simulink model "TractionSystem"  (R2019b)
settings: configuration reference "ConfigSet_TractionSystem_Reference" (kept outside this file)
model workspace (MAT data in the model file):
  Prm_TractionSystem : Simulink.Parameter (value not decoded)
  SampleTime = 0.01
symbols that are objects in the model workspace (value not decoded): Prm_TractionSystem
undefined symbols (not defined in the file): Audio, BCU, Bogie, BogieNotIsolated, DiscIntNeverNeededParam, Dynamics, EDBrakeStatus, EDBrakingEffortAchieved, EDBrakingEffortPossible, ElectricalSystem, Forward, MaxAxles, Reverse, TCMS, TCUWheelSlideControlActive, TractionContactorStatus, TractionControl, TractionEDPower, Trafo_TCU, VehicleBogieDerailed, VehicleDerailed, WheelAngularVelocity
libraries: simulink x19, LatchesLib x3, TimersLib x2, WheelSlipControl_Lib x2, simulink_extras x2, TractionLib x2
(part 2 of 2)

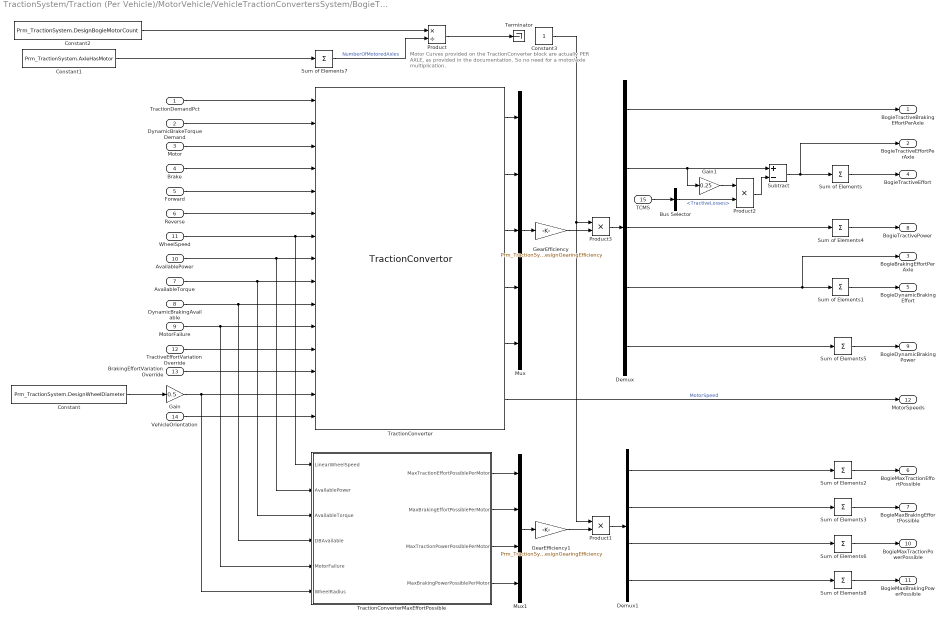
== system TractionSystem/Traction (Per Vehicle)/MotorVehicle/VehicleTractionConvertersSystem/BogieTractionConverterSystem (Per Bogie)/TractionConverterSystem ==
  note: Motor Curves provided on the TractionConverter block are actually PER AXLE, as provided in the documentation. So no need for a motor/axle multiplication.
  TractionDemandPct : Inport
  DynamicBrakeTorqueDemand : Inport  Port=2
  Motor : Inport  Port=3
  Brake : Inport  Port=4
  Forward : Inport  Port=5
  Reverse : Inport  Port=6
  AvailableTorque : Inport  Port=7
  DynamicBrakingAvailable : Inport  Port=8
  MotorFailure : Inport  Port=9
  AvailablePower : Inport  Port=10
  WheelSpeed : Inport  Port=11
  TractiveEffortVariationOverride : Inport  Port=12
  BrakingEffortVariationOverride : Inport  Port=13
  VehicleOrientation : Inport  Port=14
  TCMS : Inport  Port=15
  Bus Selector : BusSelector  OutputSignals=TractiveLosses
  Constant : Constant  Value=Prm_TractionSystem.DesignWheelDiameter
  Constant1 : Constant  Value=Prm_TractionSystem.AxleHasMotor
  Constant2 : Constant  Value=Prm_TractionSystem.DesignBogieMotorCount
  Constant3 : Constant
  Demux : Demux  Outputs=5
  Demux1 : Demux
  Gain : Gain  Gain=0.5
  Gain1 : Gain  Gain=0.25
  GearEfficiency : Gain  Gain=Prm_TractionSystem.DesignGearingEfficiency
  GearEfficiency1 : Gain  Gain=Prm_TractionSystem.DesignGearingEfficiency
  Mux : Mux  Inputs=5
  Mux1 : Mux
  Product : Product  Inputs=*/
  Product1 : Product  Inputs=**
  Product2 : Product
  Product3 : Product  Inputs=**
  Subtract : Sum  Inputs=+-
  Sum of Elements{,1..8} (9 alike) : Sum  Inputs=+
  Terminator : Terminator
  TractionConverter : TractionLib/TractionConvertor  TractionCurveInput=Curve Equations  TractionRatedTorque=Prm_TractionSystem.DesignMaxTractionTorque  TractionDesignPower=Prm_TractionSystem.DesignMaxTractionPower  TractionMotorSpeeds=[0 1]'  TractionMotorTorques=[34000 34000]'*(Prm_TractionSystem.DesignWheelDiameter/2)  VehicleTractionDataSize=2  CDMaxMotorTorque=Prm_TractionSystem.DesignMaxTractionTorque  CDMaxMotorPower=Prm_TractionSystem.DesignMaxTractionPower  TractionContourCount=4  TractionDemands=[1 2 3 4 0]  TractionDataSizes=[4 4 3 5 0]  TractionDataContours=permute(cat(3, [0 0; 1 1; 2 2; 3 3; 0 0;],[0 1; 1 2; 2.5 3; 5 4.5; 0 0;], [0 2; 2 4; 4 8; 0 0; 0 0;], [0 2.5; 1 4; 2 5; 3 9; 5 15;], [0 0; 0 0; 0 0; 0 0; 0 0;]), [3 2 1])  TractionMaximumTorques=[3 4.5 8 15 0]'  TractionMaximumPowers=[9 22.5 32 75 0]'  TractionRisingSlewRate=2e3  TractionFallingSlewRate=-5e3  BrakingCurveInput=Curve Equations  BrakingRatedTorque=Prm_TractionSystem.DesignMaxBrakingTorque  BrakingDesignPower=Prm_TractionSystem.DesignMaxBrakingPower  BrakingRampUpSpeeds=Prm_TractionSystem.BrakeFadeRampDownSpeeds  BrakingMotorSpeeds=[0 1]'  BrakingMotorTorques=[50000 50000]'*(Prm_TractionSystem.DesignWheelDiameter/2)  VehicleBrakingDataSize=2  BrakingDemands=[1 2 3 4 0]  BrakingDataSizes=[4 4 3 5 0]  BrakingDataContours=permute(cat(3, [0 0; 1 1; 2 2; 3 3; 0 0;],[0 1; 1 2; 2.5 3; 5 4.5; 0 0;], [0 2; 2 4; 4 8; 0 0; 0 0;], [0 2.5; 1 4; 2 5; 3 9; 5 15;], [0 0; 0 0; 0 0; 0 0; 0 0;]), [3 2 1])  BrakingRisingSlewRate=5e3  BrakingFallingSlewRate=-5e3  AxleHasMotor=Prm_TractionSystem.AxleHasMotor  GearRatio=Prm_TractionSystem.DesignGearingRatio
      settings: SourceProductName=Train Utilities
  TractionConverterMaxEffortPossible : Subsystem  mask{TractionRatedTorque=Prm_TractionSystem.DesignMaxTractionTorque, TractionDesignPower=Prm_TractionSystem.DesignMaxTractionPower, BrakingRatedTorque=Prm_TractionSystem.DesignMaxBrakingTorque, BrakingDesignPower=Prm_TractionSystem.DesignMaxBrakingPower, RampUpSpeeds=Prm_TractionSystem.BrakeFadeRampDownSpeeds, AxleHasMotor=Prm_TractionSystem.AxleHasMotor, GearRatio=Prm_TractionSystem.DesignGearingRatio}
      mask prompts: TractionRatedTorque "This is the constant torque for 1 motor (removing design gearing ratio and wheel diameter factors) [Nm]:"; TractionDesignPower "This is the Constant power for 100% Demand (and should be Rated Torque* Corner Motor Speed) [Nm/s]:"; BrakingRatedTorque "This is the constant torque for 1 motor (removing design gearing ratio and wheel diameter factors) [Nm]:"; BrakingDesignPower "This is the constant power for 100% Demand (and should be Rated Torque* Corner Motor Speed) [Nm/s]:"; RampUpSpeeds "This is a list of the two motor speeds between which the Dynamic Braking Avilable is ramped between 0 and 100% [rad/s]:"; GearRatio "Gear Ratio"
      mask DialogControl TractionParam Prompt: Traction
      mask DialogControl Container11 Prompt: Braking
      mask DialogControl Container9 Prompt: General
      mask DialogControl GearParam Prompt: Gearing
  BogieTractiveBrakingEffortPerAxle : Outport  PortDimensions=2
  BogieTractiveEffortPerAxle : Outport  Port=2  PortDimensions=2
  BogieBrakingEffortPerAxle : Outport  Port=3  PortDimensions=2
  BogieTractiveEffort : Outport  Port=4
  BogieDynamicBrakingEffort : Outport  Port=5
  BogieMaxTractionEffortPossible : Outport  Port=6
  BogieMaxBrakingEffortPossible : Outport  Port=7
  BogieTractivePower : Outport  Port=8
  BogieDynamicBrakingPower : Outport  Port=9
  BogieMaxTractionPowerPossible : Outport  Port=10
  BogieMaxBrakingPowerPossible : Outport  Port=11
  MotorSpeeds : Outport  Port=12
  wires:
  AvailablePower/1 -> TractionConverterMaxEffortPossible/2(AvailablePower), TractionConverter/8
  BrakingEffortVariationOverride/1 -> TractionConverter/13
  VehicleOrientation/1 -> TractionConverter/15
  MotorFailure/1 -> TractionConverterMaxEffortPossible/5(MotorFailure), TractionConverter/11
  TractiveEffortVariationOverride/1 -> TractionConverter/12
  DynamicBrakingAvailable/1 -> TractionConverterMaxEffortPossible/4(DBAvailable), TractionConverter/10
  AvailableTorque/1 -> TractionConverterMaxEffortPossible/3(AvailableTorque), TractionConverter/9
  TractionConverter/6 -> MotorSpeeds/1  "MotorSpeed"
  Constant/1 -> Gain/1
  TractionDemandPct/1 -> TractionConverter/1
  DynamicBrakeTorqueDemand/1 -> TractionConverter/2
  Motor/1 -> TractionConverter/3
  Brake/1 -> TractionConverter/4
  Forward/1 -> TractionConverter/5
  Reverse/1 -> TractionConverter/6
  WheelSpeed/1 -> TractionConverterMaxEffortPossible/1(LinearWheelSpeed), TractionConverter/7
  Sum of Elements/1 -> BogieTractiveEffort/1
  Sum of Elements1/1 -> BogieDynamicBrakingEffort/1
  Gain/1 -> TractionConverterMaxEffortPossible/6(WheelRadius), TractionConverter/14
  TractionConverterMaxEffortPossible/1(MaxTractionEffortPossiblePerMotor) -> Mux1/1
  TractionConverterMaxEffortPossible/2(MaxBrakingEffortPossiblePerMotor) -> Mux1/2
  Sum of Elements2/1 -> BogieMaxTractionEffortPossible/1
  Sum of Elements3/1 -> BogieMaxBrakingEffortPossible/1
  Sum of Elements4/1 -> BogieTractivePower/1
  Sum of Elements5/1 -> BogieDynamicBrakingPower/1
  Constant1/1 -> Sum of Elements7/1
  Sum of Elements7/1 -> Product/2  "NumberOfMotoredAxles"
  Constant2/1 -> Product/1
  Subtract/1 -> BogieTractiveEffortPerAxle/1, Sum of Elements/1
  Demux/3 -> Sum of Elements4/1
  Demux/5 -> Sum of Elements5/1
  TractionConverter/1 -> Mux/1
  TractionConverter/2 -> Mux/2
  TractionConverter/3 -> Mux/3
  TractionConverter/4 -> Mux/4
  TractionConverter/5 -> Mux/5
  Mux/1 -> GearEfficiency/1
  GearEfficiency/1 -> Product3/2
  Product3/1 -> Demux/1
  Demux/1 -> BogieTractiveBrakingEffortPerAxle/1
  Product1/1 -> Demux1/1
  Constant3/1 -> Product1/1, Product3/1
  GearEfficiency1/1 -> Product1/2
  Mux1/1 -> GearEfficiency1/1
  Demux1/1 -> Sum of Elements2/1
  Demux1/2 -> Sum of Elements3/1
  Product/1 -> Terminator/1
  TractionConverterMaxEffortPossible/3(MaxTractionPowerPossiblePerMotor) -> Mux1/3
  TractionConverterMaxEffortPossible/4(MaxBrakingPowerPossiblePerMotor) -> Mux1/4
  Demux1/4 -> Sum of Elements8/1
  Demux1/3 -> Sum of Elements6/1
  Sum of Elements8/1 -> BogieMaxBrakingPowerPossible/1
  Sum of Elements6/1 -> BogieMaxTractionPowerPossible/1
  Demux/4 -> BogieBrakingEffortPerAxle/1, Sum of Elements1/1
  TCMS/1 -> Bus Selector/1
  Bus Selector/1 -> Product2/2  "<TractiveLosses>"
  Demux/2 -> Gain1/1, Subtract/1
  Product2/1 -> Subtract/2
  Gain1/1 -> Product2/1

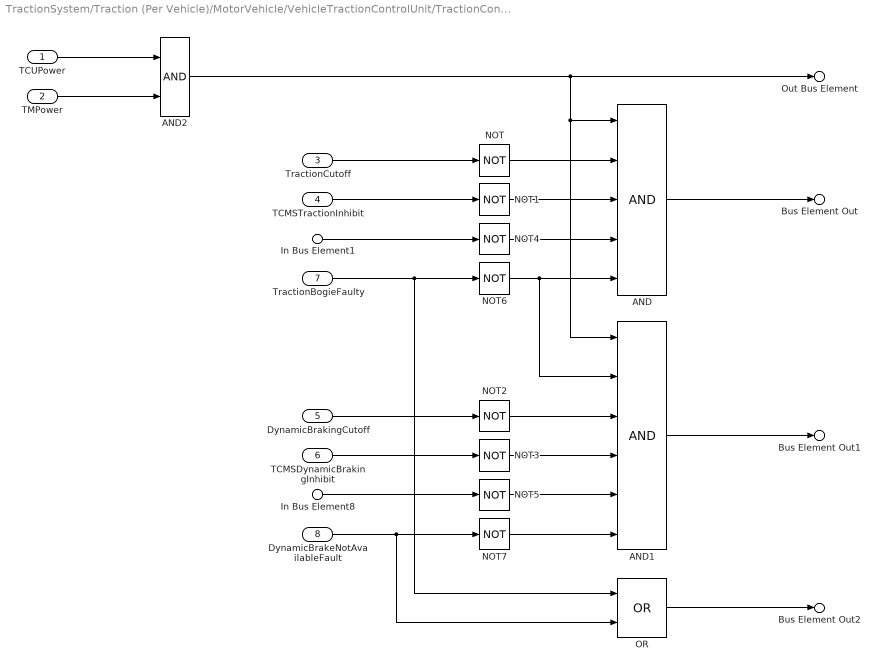
== system TractionSystem/Traction (Per Vehicle)/MotorVehicle/VehicleTractionControlUnit/TractionControl (Per Bogie)/TCUONLogic/BogieTractionBrakingAvailable ==
  TCUPower : Inport
  TMPower : Inport  Port=2
  TractionCutoff : Inport  Port=3
  TCMSTractionInhibit : Inport  Port=4
  DynamicBrakingCutoff : Inport  Port=5
  TCMSDynamicBrakingInhibit : Inport  Port=6
  TractionBogieFaulty : Inport  Port=7
  DynamicBrakeNotAvailableFault : Inport  Port=8
  In Bus Element8 : Inport  Port=9  PortName=WheelSlipSlideProtection  Element=WSPBrakeCutOut
  In Bus Element1 : Inport  Port=9  PortName=WheelSlipSlideProtection  Element=WSPTractionCutOut
  AND : Logic  Inputs=5  AllPortsSameDT=off  OutDataTypeStr=boolean
  AND1 : Logic  Inputs=6  AllPortsSameDT=off  OutDataTypeStr=boolean
  AND2 : Logic  AllPortsSameDT=off  OutDataTypeStr=boolean
  NOT{,1..7} (8 alike) : Logic  Operator=NOT  AllPortsSameDT=off  OutDataTypeStr=boolean
  OR : Logic  Operator=OR  AllPortsSameDT=off  OutDataTypeStr=boolean
  Bus Element Out : Outport  PortName=TCStatuses  Element=TractionAvailable
  Bus Element Out1 : Outport  PortName=TCStatuses  Element=EDBrakeAvailable
  Out Bus Element : Outport  PortName=TCStatuses  Element=TCUResponseStatus
  Bus Element Out2 : Outport  PortName=TCStatuses  Element=BogieFaulty
  wires:
  AND/1 -> Bus Element Out/1
  AND1/1 -> Bus Element Out1/1
  AND2/1 -> AND1/1, AND/1, Out Bus Element/1
  TractionCutoff/1 -> NOT/1
  NOT/1 -> AND/2
  TCMSTractionInhibit/1 -> NOT1/1
  NOT1/1 -> AND/3
  TCMSDynamicBrakingInhibit/1 -> NOT3/1
  DynamicBrakingCutoff/1 -> NOT2/1
  NOT3/1 -> AND1/4
  NOT2/1 -> AND1/3
  In Bus Element1/1 -> NOT4/1
  NOT4/1 -> AND/4
  In Bus Element8/1 -> NOT5/1
  NOT5/1 -> AND1/5
  TractionBogieFaulty/1 -> OR/1, NOT6/1
  NOT6/1 -> AND/5, AND1/2
  DynamicBrakeNotAvailableFault/1 -> OR/2, NOT7/1
  NOT7/1 -> AND1/6
  OR/1 -> Bus Element Out2/1
  TMPower/1 -> AND2/2
  TCUPower/1 -> AND2/1

== system TractionSystem/Traction (Per Vehicle)/MotorVehicle/VehicleTractionControlUnit/TractionControl (Per Bogie)/TCUONLogic/DirectionControl ==
  Forward : Inport
  Reverse : Inport  Port=2
  AND : Logic  AllPortsSameDT=off  OutDataTypeStr=boolean
  AND1 : Logic  AllPortsSameDT=off  OutDataTypeStr=boolean
  NOT : Logic  Operator=NOT  AllPortsSameDT=off  OutDataTypeStr=boolean
  NOT1 : Logic  Operator=NOT  AllPortsSameDT=off  OutDataTypeStr=boolean
  Bus Element Out : Outport  PortName=DirectionControl  Element=Forward
  Bus Element Out1 : Outport  PortName=DirectionControl  Element=Reverse
  wires:
  Reverse/1 -> NOT1/1, AND/2  "Reverse"
  Forward/1 -> AND1/1, NOT/1  "Forward"
  NOT/1 -> AND/1
  NOT1/1 -> AND1/2
  AND1/1 -> Bus Element Out/1
  AND/1 -> Bus Element Out1/1

== system TractionSystem/Traction (Per Vehicle)/MotorVehicle/VehicleTractionControlUnit/TractionControl (Per Bogie)/TCUONLogic/TCUControlsAssign ==
  In Bus Element : Inport  PortName=DirectionControl  Element=Forward
  In Bus Element1 : Inport  PortName=DirectionControl  Element=Reverse
  Bus Element In : Inport  Port=2  PortName=TCUStatuses  Element=TractionAvailable
  In Bus Element9 : Inport  Port=2  PortName=TCUStatuses  Element=EDBrakeAvailable
  In Bus Element2 : Inport  Port=3  PortName=TRBCommands  Element=BrakingTorqueDemand
  In Bus Element3 : Inport  Port=3  PortName=TRBCommands  Element=TractionDemandPct
  In Bus Element4 : Inport  Port=4  PortName=TRBInterlocks  Element=TractionInterlock
  In Bus Element5 : Inport  Port=4  PortName=TRBInterlocks  Element=BrakingInterlock
  Bus Creator : BusCreator  Inputs=9  OutDataTypeStr=Bus: BD_TractionSystem_Int_BogieControl  NonVirtualBus=on
  Constant1 : Constant  Value=Prm_TractionSystem.AxleHasMotor
  Data Type Conversion{1..9} (9 alike) : DataTypeConversion
  Data Type Conversion10 : DataTypeConversion  OutDataTypeStr=double
  NOT1 : Logic  Operator=NOT  AllPortsSameDT=off  OutDataTypeStr=boolean
  Product : Product
  TractionControlOut : Outport
  wires:
  Data Type Conversion6/1 -> Bus Creator/8  "TractionTorqueAvailable"
  In Bus Element4/1 -> Data Type Conversion2/1
  Data Type Conversion1/1 -> Bus Creator/4  "Braking"
  Data Type Conversion8/1 -> Bus Creator/9  "DynamicBrakeAvailable"
  Constant1/1 -> Product/1
  Data Type Conversion2/1 -> Bus Creator/3  "Powering"
  Bus Element In/1 -> Data Type Conversion6/1, Data Type Conversion10/1
  In Bus Element5/1 -> Data Type Conversion1/1
  Bus Creator/1 -> TractionControlOut/1
  In Bus Element3/1 -> Data Type Conversion9/1
  In Bus Element2/1 -> Data Type Conversion7/1
  In Bus Element1/1 -> Data Type Conversion4/1
  Data Type Conversion4/1 -> Bus Creator/6  "Reverse"
  Data Type Conversion3/1 -> Bus Creator/5  "Forward"
  In Bus Element/1 -> Data Type Conversion3/1
  NOT1/1 -> Data Type Conversion5/1
  Data Type Conversion5/1 -> Bus Creator/7  "MotorNotAvailable"
  Product/1 -> NOT1/1
  Data Type Conversion10/1 -> Product/2
  In Bus Element9/1 -> Data Type Conversion8/1
  Data Type Conversion7/1 -> Bus Creator/2  "DynamicBrakeTorqueDemand"
  Data Type Conversion9/1 -> Bus Creator/1  "TractionDemandPct"

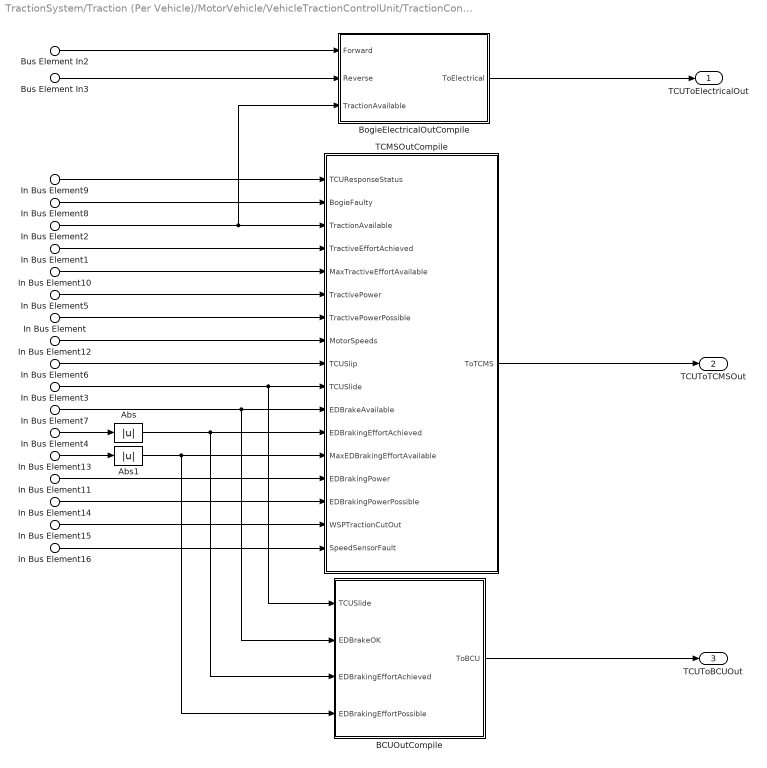
== system TractionSystem/Traction (Per Vehicle)/MotorVehicle/VehicleTractionControlUnit/TractionControl (Per Bogie)/TCUONLogic/TCUOutputsAssign ==
  Bus Element In2 : Inport  PortName=DirectionControlOut  Element=Forward
  Bus Element In3 : Inport  PortName=DirectionControlOut  Element=Reverse
  In Bus Element1 : Inport  Port=2  PortName=TractionConverterOut  Element=BogieTractiveEffort
  In Bus Element4 : Inport  Port=2  PortName=TractionConverterOut  Element=BogieDynamicBrakingEffort
  In Bus Element10 : Inport  Port=2  PortName=TractionConverterOut  Element=BogieMaxTractionEffortPossible
  In Bus Element5 : Inport  Port=2  PortName=TractionConverterOut  Element=BogieTractivePower
  In Bus Element11 : Inport  Port=2  PortName=TractionConverterOut  Element=BogieDynamicBrakingPower
  In Bus Element12 : Inport  Port=2  PortName=TractionConverterOut  Element=BogieMotorSpeeds
  In Bus Element13 : Inport  Port=2  PortName=TractionConverterOut  Element=BogieMaxBrakingEffortPossible
  In Bus Element : Inport  Port=2  PortName=TractionConverterOut  Element=BogieMaxTractionPowerPossible
  In Bus Element14 : Inport  Port=2  PortName=TractionConverterOut  Element=BogieMaxBrakingPowerPossible
  In Bus Element2 : Inport  Port=3  PortName=TCStatuses  Element=TractionAvailable
  In Bus Element7 : Inport  Port=3  PortName=TCStatuses  Element=EDBrakeAvailable
  In Bus Element9 : Inport  Port=3  PortName=TCStatuses  Element=TCUResponseStatus
  In Bus Element8 : Inport  Port=3  PortName=TCStatuses  Element=BogieFaulty
  In Bus Element3 : Inport  Port=4  PortName=WheelSlipSlideProtection  Element=TCUSlide
  In Bus Element6 : Inport  Port=4  PortName=WheelSlipSlideProtection  Element=TCUSlip
  In Bus Element15 : Inport  Port=4  PortName=WheelSlipSlideProtection  Element=WSPTractionCutOut
  In Bus Element16 : Inport  Port=5  PortName=Sensor  Element=SpeedSensorFault
  Abs : Abs
  Abs1 : Abs
  BCUOutCompile : Subsystem
  BogieElectricalOutCompile : Subsystem
  TCMSOutCompile : Subsystem
  TCUToElectricalOut : Outport
  TCUToTCMSOut : Outport  Port=2
  TCUToBCUOut : Outport  Port=3
  wires:
  TCMSOutCompile/1(ToTCMS) -> TCUToTCMSOut/1
  In Bus Element7/1 -> BCUOutCompile/2(EDBrakeOK), TCMSOutCompile/11(EDBrakeAvailable)
  In Bus Element4/1 -> Abs/1
  In Bus Element1/1 -> TCMSOutCompile/4(TractiveEffortAchieved)
  BCUOutCompile/1(ToBCU) -> TCUToBCUOut/1
  BogieElectricalOutCompile/1(ToElectrical) -> TCUToElectricalOut/1
  In Bus Element10/1 -> TCMSOutCompile/5(MaxTractiveEffortAvailable)
  In Bus Element13/1 -> Abs1/1
  In Bus Element3/1 -> BCUOutCompile/1(TCUSlide), TCMSOutCompile/10(TCUSlide)
  Bus Element In2/1 -> BogieElectricalOutCompile/1(Forward)
  In Bus Element2/1 -> BogieElectricalOutCompile/3(TractionAvailable), TCMSOutCompile/3(TractionAvailable)
  In Bus Element6/1 -> TCMSOutCompile/9(TCUSlip)
  Abs/1 -> BCUOutCompile/3(EDBrakingEffortAchieved), TCMSOutCompile/12(EDBrakingEffortAchieved)
  Abs1/1 -> BCUOutCompile/4(EDBrakingEffortPossible), TCMSOutCompile/13(MaxEDBrakingEffortAvailable)
  In Bus Element9/1 -> TCMSOutCompile/1(TCUResponseStatus)
  Bus Element In3/1 -> BogieElectricalOutCompile/2(Reverse)
  In Bus Element11/1 -> TCMSOutCompile/14(EDBrakingPower)
  In Bus Element5/1 -> TCMSOutCompile/6(TractivePower)
  In Bus Element12/1 -> TCMSOutCompile/8(MotorSpeeds)
  In Bus Element/1 -> TCMSOutCompile/7(TractivePowerPossible)
  In Bus Element14/1 -> TCMSOutCompile/15(EDBrakingPowerPossible)
  In Bus Element8/1 -> TCMSOutCompile/2(BogieFaulty)
  In Bus Element15/1 -> TCMSOutCompile/16(WSPTractionCutOut)
  In Bus Element16/1 -> TCMSOutCompile/17(SpeedSensorFault)

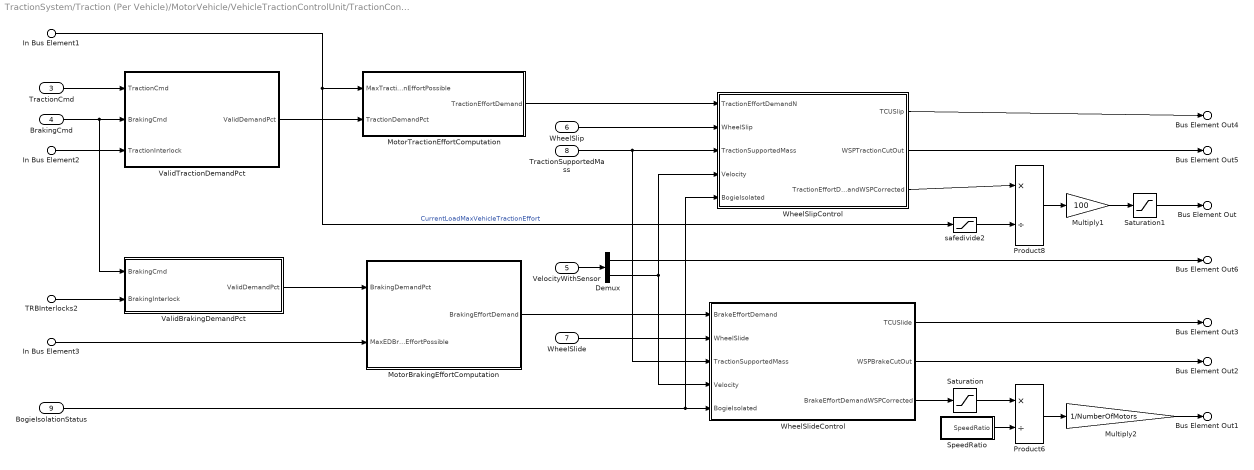
== system TractionSystem/Traction (Per Vehicle)/MotorVehicle/VehicleTractionControlUnit/TractionControl (Per Bogie)/TCUONLogic/TractionBrakingDemandControl ==
  In Bus Element1 : Inport  PortName=TCOut  Element=BogieMaxTractionEffortPossible
  In Bus Element3 : Inport  PortName=TCOut  Element=BogieMaxBrakingEffortPossible
  TRBInterlocks2 : Inport  Port=2  PortName=TRBInterlocks  Element=BrakingInterlock
  In Bus Element2 : Inport  Port=2  PortName=TRBInterlocks  Element=TractionInterlock
  TractionCmd : Inport  Port=3
  BrakingCmd : Inport  Port=4
  VelocityWithSensor : Inport  Port=5
  WheelSlip : Inport  Port=6
  WheelSlide : Inport  Port=7
  TractionSupportedMass : Inport  Port=8
  BogieIsolationStatus : Inport  Port=9
  Demux : Demux  Outputs=2
  MotorBrakingEffortComputation : Subsystem
  MotorTractionEffortComputation : Subsystem
  Multiply1 : Gain  Gain=100
  Multiply2 : Gain  Gain=1/NumberOfMotors
  Product6 : Product  Inputs=*/
  Product8 : Product  Inputs=*/
  Saturation : Saturate  UpperLimit=inf  LowerLimit=0
  Saturation1 : Saturate  UpperLimit=100  LowerLimit=0
  SpeedRatio : Subsystem
  ValidBrakingDemandPct : Subsystem
  ValidTractionDemandPct : Subsystem
  WheelSlideControl : Subsystem
  WheelSlipControl : Subsystem
  safedivide2 : Saturate  UpperLimit=1e8  LowerLimit=eps
  Bus Element Out2 : Outport  PortName=WheelSlipSlideProtection  Element=WSPBrakeCutOut
  Bus Element Out3 : Outport  PortName=WheelSlipSlideProtection  Element=TCUSlide
  Bus Element Out4 : Outport  PortName=WheelSlipSlideProtection  Element=TCUSlip
  Bus Element Out5 : Outport  PortName=WheelSlipSlideProtection  Element=WSPTractionCutOut
  Bus Element Out6 : Outport  Port=2  PortName=Sensor  Element=SpeedSensorFault
  Bus Element Out : Outport  Port=3  PortName=TRBCommands  Element=TractionDemandPct
  Bus Element Out1 : Outport  Port=3  PortName=TRBCommands  Element=BrakingTorqueDemand
  wires:
  Product8/1 -> Multiply1/1
  Product6/1 -> Multiply2/1
  Saturation/1 -> Product6/1
  WheelSlideControl/3(BrakeEffortDemandWSPCorrected) -> Saturation/1
  MotorTractionEffortComputation/1(TractionEffortDemand) -> WheelSlipControl/1(TractionEffortDemandN)
  SpeedRatio/1(SpeedRatio) -> Product6/2
  WheelSlide/1 -> WheelSlideControl/2(WheelSlide)
  WheelSlideControl/2(WSPBrakeCutOut) -> Bus Element Out2/1
  WheelSlideControl/1(TCUSlide) -> Bus Element Out3/1
  WheelSlipControl/1("TCUSlip ") -> Bus Element Out4/1
  WheelSlip/1 -> WheelSlipControl/2(WheelSlip)
  WheelSlipControl/3(TractionEffortDemandWSPCorrected) -> Product8/1
  In Bus Element1/1 -> safedivide2/1, MotorTractionEffortComputation/1(MaxTractionEffortPossible)  "CurrentLoadMaxVehicleTractionEffort"
  Multiply1/1 -> Saturation1/1
  BrakingCmd/1 -> ValidTractionDemandPct/2(BrakingCmd), ValidBrakingDemandPct/1(BrakingCmd)
  ValidBrakingDemandPct/1(ValidDemandPct) -> MotorBrakingEffortComputation/1(BrakingDemandPct)
  TractionCmd/1 -> ValidTractionDemandPct/1(TractionCmd)
  ValidTractionDemandPct/1(ValidDemandPct) -> MotorTractionEffortComputation/2(TractionDemandPct)
  MotorBrakingEffortComputation/1(BrakingEffortDemand) -> WheelSlideControl/1(BrakeEffortDemand)
  safedivide2/1 -> Product8/2
  Saturation1/1 -> Bus Element Out/1
  In Bus Element3/1 -> MotorBrakingEffortComputation/2(MaxEDBrakingEffortPossible)
  In Bus Element2/1 -> ValidTractionDemandPct/3(TractionInterlock)
  TRBInterlocks2/1 -> ValidBrakingDemandPct/2(BrakingInterlock)
  TractionSupportedMass/1 -> WheelSlideControl/3(TractionSupportedMass), WheelSlipControl/3(TractionSupportedMass)
  Multiply2/1 -> Bus Element Out1/1
  WheelSlipControl/2(WSPTractionCutOut) -> Bus Element Out5/1
  Demux/2 -> WheelSlipControl/4(Velocity), WheelSlideControl/4(Velocity)
  VelocityWithSensor/1 -> Demux/1
  Demux/1 -> Bus Element Out6/1
  BogieIsolationStatus/1 -> WheelSlipControl/5(BogieIsolated), WheelSlideControl/5(BogieIsolated)

== system TractionSystem/Traction (Per Vehicle)/MotorVehicle/VehicleTractionControlUnit/TractionControl (Per Bogie)/TCUONLogic/TractionBrakingInterlocks ==
  Bus Element In2 : Inport  PortName=DirectionControlOut  Element=Forward
  Bus Element In3 : Inport  PortName=DirectionControlOut  Element=Reverse
  TractionAuthorisation : Inport  Port=2
  TractionActive : Inport  Port=3
  NoEmergencyBrakeActive : Inport  Port=4
  Constant : Constant  Value=true  OutDataTypeStr=boolean
  Constant1 : Constant  Value=EBdeactivateED
  Data Type Conversion3 : DataTypeConversion
  Data Type Conversion4 : DataTypeConversion
  OR1 : Logic  Operator=OR  AllPortsSameDT=off  OutDataTypeStr=boolean
  Switch : Switch  Criteria=u2 > Threshold
  Vector Concatenate : Concatenate  NumInputs=3
  Vector Concatenate1 : Concatenate
  and : Logic  AllPortsSameDT=off  OutDataTypeStr=boolean
  and1 : Logic  Inputs=1  AllPortsSameDT=off  OutDataTypeStr=boolean
  and5 : Logic  Inputs=1  AllPortsSameDT=off  OutDataTypeStr=boolean
  Bus Element Out : Outport  PortName=TRBInterlocks  Element=TractionInterlock
  Bus Element Out1 : Outport  PortName=TRBInterlocks  Element=BrakingInterlock
  wires:
  and/1 -> Data Type Conversion3/1
  Data Type Conversion3/1 -> Bus Element Out/1  "TractionInterlock"
  Data Type Conversion4/1 -> Bus Element Out1/1  "BrakingInterlock"
  and1/1 -> and/1, Data Type Conversion4/1
  Vector Concatenate/1 -> and5/1
  Bus Element In2/1 -> OR1/1
  Bus Element In3/1 -> OR1/2
  OR1/1 -> Vector Concatenate1/1
  TractionActive/1 -> Vector Concatenate/2
  NoEmergencyBrakeActive/1 -> Switch/1, Vector Concatenate/1
  and5/1 -> and/2
  Vector Concatenate1/1 -> and1/1
  Switch/1 -> Vector Concatenate1/2
  Constant/1 -> Switch/3
  Constant1/1 -> Switch/2
  TractionAuthorisation/1 -> Vector Concatenate/3

== system TractionSystem/Traction (Per Vehicle)/MotorVehicle/VehicleTractionConvertersSystem/BogieTractionConverterSystem (Per Bogie)/TractionConverterSystem/TractionConverterMaxEffortPossible ==
  LinearWheelSpeed : Inport
  AvailablePower : Inport  Port=2
  AvailableTorque : Inport  Port=3
  DBAvailable : Inport  Port=4
  MotorFailure : Inport  Port=5
  WheelRadius : Inport  Port=6
  Assignment : Assignment  DiagnosticForDimensions=Warning  IndexOptions=Assign all  Indices=1  OutputSizes=1
  Constant : Constant  Value=AxleHasMotor
  MotorVehicle : Subsystem
  MaxTractionEffortPossiblePerMotor : Outport
  MaxBrakingEffortPossiblePerMotor : Outport  Port=2
  MaxTractionPowerPossiblePerMotor : Outport  Port=3
  MaxBrakingPowerPossiblePerMotor : Outport  Port=4
  wires:
  LinearWheelSpeed/1 -> Assignment/2
  AvailablePower/1 -> MotorVehicle/3(AvailablePower)
  AvailableTorque/1 -> MotorVehicle/4(AvailableTorque)
  WheelRadius/1 -> MotorVehicle/5(WheelRadius)
  MotorVehicle/1(MaximumTractionEffortPossible) -> MaxTractionEffortPossiblePerMotor/1
  MotorVehicle/2(MaxBrakingEffortPossible) -> MaxBrakingEffortPossiblePerMotor/1
  Constant/1 -> Assignment/1, MotorVehicle/1(AxleHasMotor)
  MotorFailure/1 -> MotorVehicle/6(MotorFailure)
  DBAvailable/1 -> MotorVehicle/7(DBAvailable)
  MotorVehicle/4(MaxBrakingPowerPossible) -> MaxBrakingPowerPossiblePerMotor/1
  MotorVehicle/3(MaxTractionPowerPossible) -> MaxTractionPowerPossiblePerMotor/1
  Assignment/1 -> MotorVehicle/2(LinearWheelSpeed)

== system TractionSystem/Traction (Per Vehicle)/MotorVehicle/VehicleTractionControlUnit/TractionControl (Per Bogie)/TCUONLogic/TCUOutputsAssign/BCUOutCompile ==
  TCUSlide : Inport
  EDBrakeOK : Inport  Port=2
  EDBrakingEffortAchieved : Inport  Port=3
  EDBrakingEffortPossible : Inport  Port=4
  Bus Assignment1 : BusAssignment  AssignedSignals=TCUWheelSlideControlActive,EDBrakeStatus,EDBrakingEffortAchieved,EDBrakingEffortPossible
  Constant1 : Constant  Value=0  OutDataTypeStr=Bus: BD_TractionSystem_Out_Vehicle_BCU_Bogie
  Data Type Conversion : DataTypeConversion
  ToBCU : Outport
  wires:
  Bus Assignment1/1 -> ToBCU/1  "ToBCU"
  Constant1/1 -> Bus Assignment1/1
  EDBrakeOK/1 -> Bus Assignment1/3
  EDBrakingEffortPossible/1 -> Bus Assignment1/5  "TotalEDBrakingEffortPossible"
  EDBrakingEffortAchieved/1 -> Bus Assignment1/4  "TotalEDBrakingEffortAchieved"
  TCUSlide/1 -> Data Type Conversion/1
  Data Type Conversion/1 -> Bus Assignment1/2

== system TractionSystem/Traction (Per Vehicle)/MotorVehicle/VehicleTractionControlUnit/TractionControl (Per Bogie)/TCUONLogic/TCUOutputsAssign/BogieElectricalOutCompile ==
  Forward : Inport
  Reverse : Inport  Port=2
  TractionAvailable : Inport  Port=3
  Bus Assignment1 : BusAssignment  AssignedSignals=Forward,Reverse,BogieNotIsolated
  Constant4 : Constant  Value=0  OutDataTypeStr=Bus: BD_TractionSystem_Out_Vehicle_ElectricalSystem_Bogie
  Data Type Conversion : DataTypeConversion  OutDataTypeStr=boolean
  Data Type Conversion1 : DataTypeConversion  OutDataTypeStr=boolean
  Data Type Conversion2 : DataTypeConversion  OutDataTypeStr=boolean
  ToElectrical : Outport
  wires:
  Reverse/1 -> Data Type Conversion1/1
  Forward/1 -> Data Type Conversion/1
  Constant4/1 -> Bus Assignment1/1
  Bus Assignment1/1 -> ToElectrical/1  "ToElectrical"
  TractionAvailable/1 -> Data Type Conversion2/1
  Data Type Conversion/1 -> Bus Assignment1/2
  Data Type Conversion1/1 -> Bus Assignment1/3
  Data Type Conversion2/1 -> Bus Assignment1/4

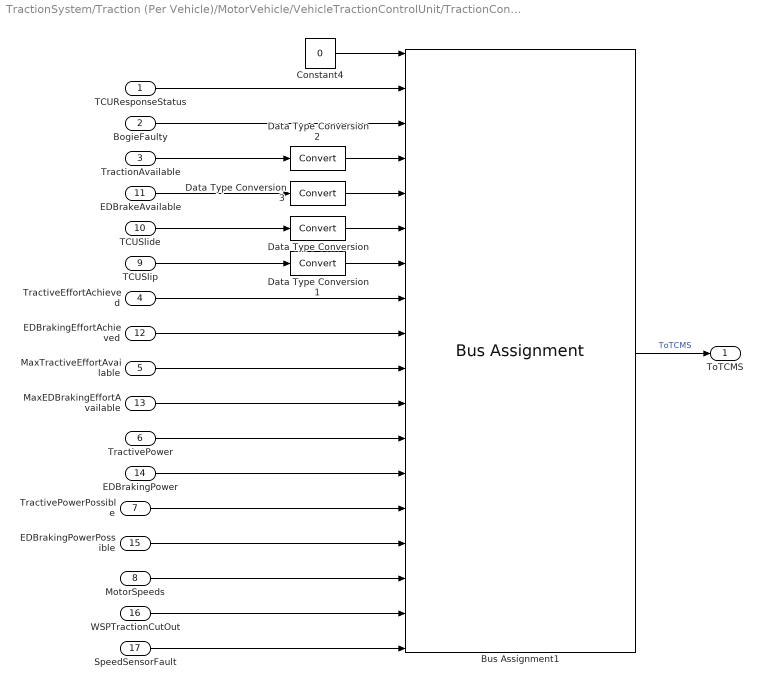
== system TractionSystem/Traction (Per Vehicle)/MotorVehicle/VehicleTractionControlUnit/TractionControl (Per Bogie)/TCUONLogic/TCUOutputsAssign/TCMSOutCompile ==
  TCUResponseStatus : Inport
  BogieFaulty : Inport  Port=2
  TractionAvailable : Inport  Port=3
  TractiveEffortAchieved : Inport  Port=4
  MaxTractiveEffortAvailable : Inport  Port=5
  TractivePower : Inport  Port=6
  TractivePowerPossible : Inport  Port=7
  MotorSpeeds : Inport  Port=8
  TCUSlip : Inport  Port=9
  TCUSlide : Inport  Port=10
  EDBrakeAvailable : Inport  Port=11
  EDBrakingEffortAchieved : Inport  Port=12
  MaxEDBrakingEffortAvailable : Inport  Port=13
  EDBrakingPower : Inport  Port=14
  EDBrakingPowerPossible : Inport  Port=15
  WSPTractionCutOut : Inport  Port=16
  SpeedSensorFault : Inport  Port=17
  Bus Assignment1 : BusAssignment  AssignedSignals=TCUStatus,BogieFaulty,TractionNotIsolated,EDBrakeNotIsolated,TCUSlideDetected,TCUSlipDetected,TractiveEffortAchieved,EDBrakingEffortAchieved,TractiveEffortPossible,EDBrakingEffortPossible,TractionPower,EDBrakingPower,TractivePowerPossible,EDBrakingPowerPossible,MotorSpeeds,WSPTractionCutout,SpeedSensorFault
  Constant4 : Constant  Value=0  OutDataTypeStr=Bus: BD_TractionSystem_Out_Vehicle_TCMS_Bogie
  Data Type Conversion{,1..3} (4 alike) : DataTypeConversion
  ToTCMS : Outport
  wires:
  TCUSlide/1 -> Data Type Conversion/1
  Bus Assignment1/1 -> ToTCMS/1  "ToTCMS"
  Constant4/1 -> Bus Assignment1/1
  TCUSlip/1 -> Data Type Conversion1/1
  TCUResponseStatus/1 -> Bus Assignment1/2
  TractionAvailable/1 -> Data Type Conversion2/1
  Data Type Conversion2/1 -> Bus Assignment1/4
  Data Type Conversion/1 -> Bus Assignment1/6
  Data Type Conversion1/1 -> Bus Assignment1/7
  TractiveEffortAchieved/1 -> Bus Assignment1/8
  EDBrakingEffortAchieved/1 -> Bus Assignment1/9
  MaxTractiveEffortAvailable/1 -> Bus Assignment1/10
  MaxEDBrakingEffortAvailable/1 -> Bus Assignment1/11
  EDBrakingPower/1 -> Bus Assignment1/13
  TractivePower/1 -> Bus Assignment1/12
  MotorSpeeds/1 -> Bus Assignment1/16
  TractivePowerPossible/1 -> Bus Assignment1/14
  EDBrakingPowerPossible/1 -> Bus Assignment1/15
  Data Type Conversion3/1 -> Bus Assignment1/5
  EDBrakeAvailable/1 -> Data Type Conversion3/1
  BogieFaulty/1 -> Bus Assignment1/3
  WSPTractionCutOut/1 -> Bus Assignment1/17
  SpeedSensorFault/1 -> Bus Assignment1/18

== system TractionSystem/Traction (Per Vehicle)/MotorVehicle/VehicleTractionControlUnit/TractionControl (Per Bogie)/TCUONLogic/TractionBrakingDemandControl/MotorBrakingEffortComputation ==
  BrakingDemandPct : Inport
  MaxEDBrakingEffortPossible : Inport  Port=2
  Multiply : Gain  Gain=0.01
  Product : Product
  BrakingEffortDemand : Outport
  wires:
  Product/1 -> BrakingEffortDemand/1
  Multiply/1 -> Product/2
  BrakingDemandPct/1 -> Multiply/1
  MaxEDBrakingEffortPossible/1 -> Product/1

== system TractionSystem/Traction (Per Vehicle)/MotorVehicle/VehicleTractionControlUnit/TractionControl (Per Bogie)/TCUONLogic/TractionBrakingDemandControl/MotorTractionEffortComputation ==
  MaxTractionEffortPossible : Inport
  TractionDemandPct : Inport  Port=2
  Multiply : Gain  Gain=0.01
  Product4 : Product
  TractionEffortDemand : Outport
  wires:
  Product4/1 -> TractionEffortDemand/1
  MaxTractionEffortPossible/1 -> Product4/1
  Multiply/1 -> Product4/2
  TractionDemandPct/1 -> Multiply/1

== system TractionSystem/Traction (Per Vehicle)/MotorVehicle/VehicleTractionControlUnit/TractionControl (Per Bogie)/TCUONLogic/TractionBrakingDemandControl/SpeedRatio ==
  Constant1 : Constant  Value=GearRatio
  Constant2 : Constant  Value=WheelDiam
  Multiply1 : Gain  Gain=0.5
  Pmax/v1 : Product  Inputs=*/
  safedivide1 : Saturate  UpperLimit=1e6  LowerLimit=eps
  safedivide2 : Saturate  UpperLimit=1e6  LowerLimit=eps
  SpeedRatio : Outport
  wires:
  safedivide1/1 -> Pmax/v1/2
  Pmax/v1/1 -> safedivide2/1
  Multiply1/1 -> safedivide1/1
  Constant2/1 -> Multiply1/1
  Constant1/1 -> Pmax/v1/1
  safedivide2/1 -> SpeedRatio/1

== system TractionSystem/Traction (Per Vehicle)/MotorVehicle/VehicleTractionControlUnit/TractionControl (Per Bogie)/TCUONLogic/TractionBrakingDemandControl/ValidBrakingDemandPct ==
  BrakingCmd : Inport
  BrakingInterlock : Inport  Port=2
  Constant : Constant  Value=0
  Switch : Switch  Criteria=u2 > Threshold
  ValidDemandPct : Outport
  wires:
  BrakingCmd/1 -> Switch/1
  Switch/1 -> ValidDemandPct/1  "BrakingDemandPct"
  BrakingInterlock/1 -> Switch/2
  Constant/1 -> Switch/3

== system TractionSystem/Traction (Per Vehicle)/MotorVehicle/VehicleTractionControlUnit/TractionControl (Per Bogie)/TCUONLogic/TractionBrakingDemandControl/ValidTractionDemandPct ==
  TractionCmd : Inport
  BrakingCmd : Inport  Port=2
  TractionInterlock : Inport  Port=3
  Compare To Zero : simulink/Logic and Bit Operations/Compare To Zero  relop=>  OutDataTypeStr=boolean
  Constant : Constant  Value=0
  NOT : Logic  Operator=NOT  AllPortsSameDT=off  OutDataTypeStr=boolean
  OR : Logic  Operator=OR  AllPortsSameDT=off  OutDataTypeStr=boolean
  Switch : Switch  Criteria=u2 > Threshold
  ValidDemandPct : Outport
  wires:
  BrakingCmd/1 -> Compare To Zero/1
  NOT/1 -> OR/1
  Switch/1 -> ValidDemandPct/1  "ValidDemandPct"
  TractionInterlock/1 -> OR/2
  TractionCmd/1 -> Switch/1
  Compare To Zero/1 -> NOT/1
  OR/1 -> Switch/2
  Constant/1 -> Switch/3

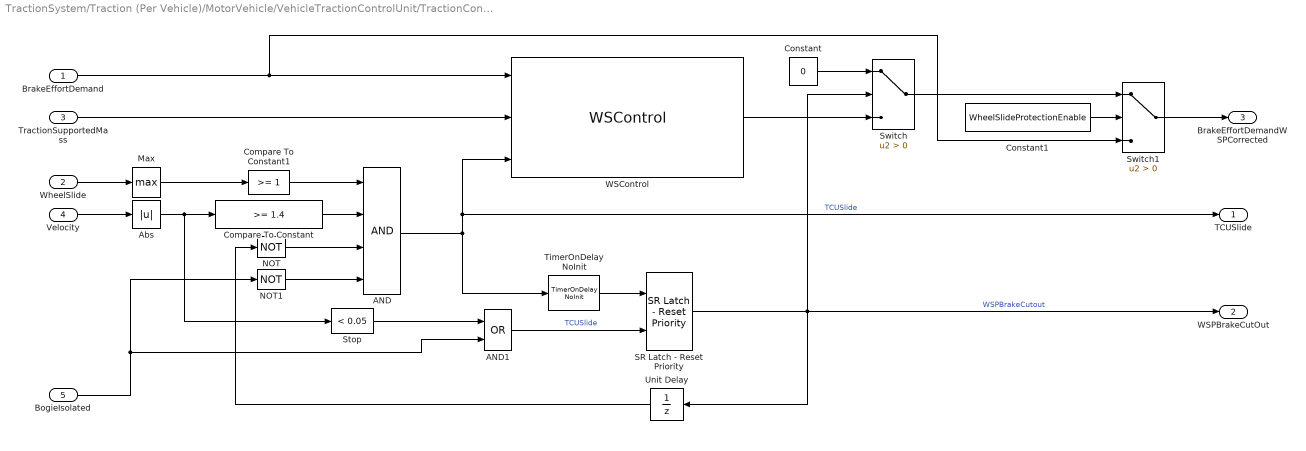
== system TractionSystem/Traction (Per Vehicle)/MotorVehicle/VehicleTractionControlUnit/TractionControl (Per Bogie)/TCUONLogic/TractionBrakingDemandControl/WheelSlideControl ==
  BrakeEffortDemand : Inport
  WheelSlide : Inport  Port=2
  TractionSupportedMass : Inport  Port=3
  Velocity : Inport  Port=4
  BogieIsolated : Inport  Port=5
  AND : Logic  Inputs=4  AllPortsSameDT=off  OutDataTypeStr=boolean
  AND1 : Logic  Operator=OR  AllPortsSameDT=off  OutDataTypeStr=boolean
  Abs : Abs
  Compare To Constant : simulink/Logic and Bit Operations/Compare To Constant  relop=>=  const=1.4  OutDataTypeStr=boolean
  Compare To Constant1 : simulink/Logic and Bit Operations/Compare To Constant  relop=>=  const=1  OutDataTypeStr=boolean
  Constant : Constant  Value=0
  Constant1 : Constant  Value=WheelSlideProtectionEnable
  Max : MinMax  Function=max
  NOT : Logic  Operator=NOT  AllPortsSameDT=off  OutDataTypeStr=boolean
  NOT1 : Logic  Operator=NOT  AllPortsSameDT=off  OutDataTypeStr=boolean
  SR Latch - Reset Priority : LatchesLib/SR Latch - Reset Priority  initial_condition=0
      settings: SourceProductName=Latches
  Stop : simulink/Logic and Bit Operations/Compare To Constant  relop=<  const=0.05  OutDataTypeStr=boolean
  Switch : Switch  Criteria=u2 > Threshold
  Switch1 : Switch  Criteria=u2 > Threshold
  TimerOnDelay NoInit : TimersLib/TimerOnDelay NoInit  UpperSaturationLimit=MaxSlideTime  OutputTime=off  SampleTime=-1
      settings: SourceProductName=Sydac Utilities
  Unit Delay : UnitDelay  SampleTime=-1  HasFrameUpgradeWarning=on
  WSControl : WheelSlipControl_Lib/WSControl  JerkLim=JerkLimit
  TCUSlide : Outport
  WSPBrakeCutOut : Outport  Port=2
  BrakeEffortDemandWSPCorrected : Outport  Port=3
  wires:
  AND/1 -> TimerOnDelay NoInit/1, WSControl/3, TCUSlide/1  "TCUSlide"
  TractionSupportedMass/1 -> WSControl/2
  WSControl/1 -> Switch/3
  Constant/1 -> Switch/1
  BrakeEffortDemand/1 -> Switch1/3, WSControl/1
  Velocity/1 -> Abs/1
  WheelSlide/1 -> Max/1
  Abs/1 -> Stop/1, Compare To Constant/1
  Compare To Constant/1 -> AND/2
  Max/1 -> Compare To Constant1/1
  Compare To Constant1/1 -> AND/1
  NOT/1 -> AND/3
  TimerOnDelay NoInit/1 -> SR Latch - Reset Priority/1
  Stop/1 -> AND1/1
  SR Latch - Reset Priority/1 -> Switch/2, WSPBrakeCutOut/1, Unit Delay/1  "WSPBrakeCutout"
  Unit Delay/1 -> NOT/1
  Constant1/1 -> Switch1/2
  Switch/1 -> Switch1/1
  Switch1/1 -> BrakeEffortDemandWSPCorrected/1
  NOT1/1 -> AND/4
  BogieIsolated/1 -> AND1/2, NOT1/1
  AND1/1 -> SR Latch - Reset Priority/2  "TCUSlide"

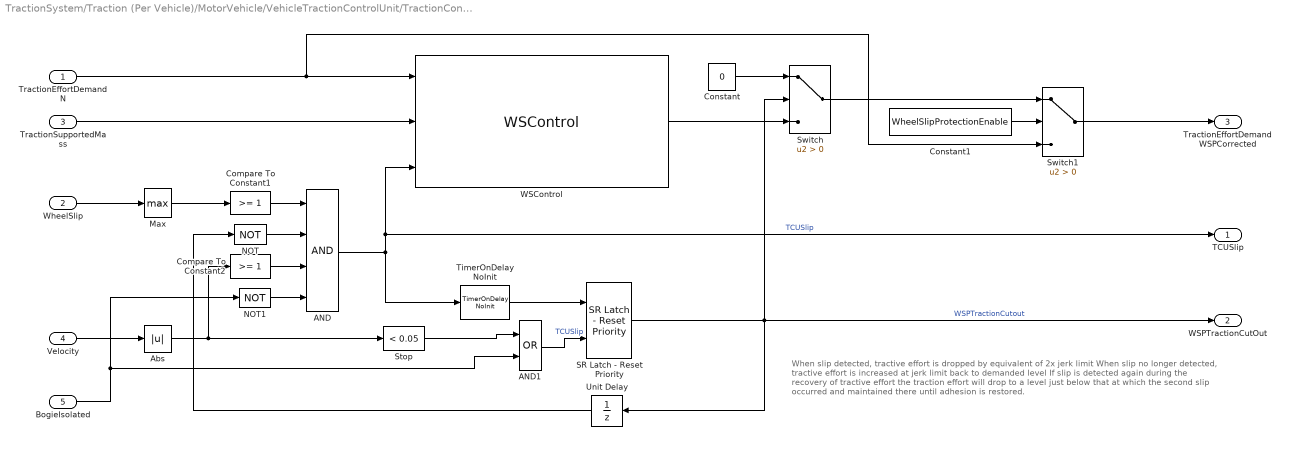
== system TractionSystem/Traction (Per Vehicle)/MotorVehicle/VehicleTractionControlUnit/TractionControl (Per Bogie)/TCUONLogic/TractionBrakingDemandControl/WheelSlipControl ==
  note: When slip detected, tractive effort is dropped by equivalent of 2x jerk limit
      | When slip no longer detected, tractive effort is increased at jerk limit back to demanded level
      | If slip is detected again during the recovery of tractive effort the traction effort will drop to a level just below that at which the second slip occurred and maintained there until adhesion is restored.
  TractionEffortDemandN : Inport
  WheelSlip : Inport  Port=2
  TractionSupportedMass : Inport  Port=3
  Velocity : Inport  Port=4
  BogieIsolated : Inport  Port=5
  AND : Logic  Inputs=4  AllPortsSameDT=off  OutDataTypeStr=boolean
  AND1 : Logic  Operator=OR  AllPortsSameDT=off  OutDataTypeStr=boolean
  Abs : Abs
  Compare To Constant1 : simulink/Logic and Bit Operations/Compare To Constant  relop=>=  const=1  OutDataTypeStr=boolean
  Compare To Constant2 : simulink/Logic and Bit Operations/Compare To Constant  relop=>=  const=1  OutDataTypeStr=boolean
  Constant : Constant  Value=0
  Constant1 : Constant  Value=WheelSlipProtectionEnable
  Max : MinMax  Function=max
  NOT : Logic  Operator=NOT  AllPortsSameDT=off  OutDataTypeStr=boolean
  NOT1 : Logic  Operator=NOT  AllPortsSameDT=off  OutDataTypeStr=boolean
  SR Latch - Reset Priority : LatchesLib/SR Latch - Reset Priority  initial_condition=0
      settings: SourceProductName=Latches
  Stop : simulink/Logic and Bit Operations/Compare To Constant  relop=<  const=0.05  OutDataTypeStr=boolean
  Switch : Switch  Criteria=u2 > Threshold
  Switch1 : Switch  Criteria=u2 > Threshold
  TimerOnDelay NoInit : TimersLib/TimerOnDelay NoInit  UpperSaturationLimit=MaxSlipTime  OutputTime=off  SampleTime=-1
      settings: SourceProductName=Sydac Utilities
  Unit Delay : UnitDelay  SampleTime=-1  HasFrameUpgradeWarning=on
  WSControl : WheelSlipControl_Lib/WSControl  JerkLim=JerkLimit
  "TCUSlip " : Outport
  WSPTractionCutOut : Outport  Port=2
  TractionEffortDemandWSPCorrected : Outport  Port=3
  wires:
  WheelSlip/1 -> Max/1
  TractionEffortDemandN/1 -> Switch1/3, WSControl/1
  WSControl/1 -> Switch/3
  TractionSupportedMass/1 -> WSControl/2
  Max/1 -> Compare To Constant1/1
  Velocity/1 -> Abs/1
  AND/1 -> WSControl/3, "TCUSlip "/1, TimerOnDelay NoInit/1  "TCUSlip"
  Constant/1 -> Switch/1
  Unit Delay/1 -> NOT/1
  Stop/1 -> AND1/1
  TimerOnDelay NoInit/1 -> SR Latch - Reset Priority/1
  SR Latch - Reset Priority/1 -> WSPTractionCutOut/1, Unit Delay/1, Switch/2  "WSPTractionCutout"
  Switch/1 -> Switch1/1
  Compare To Constant1/1 -> AND/1
  NOT/1 -> AND/2
  Switch1/1 -> TractionEffortDemandWSPCorrected/1
  Constant1/1 -> Switch1/2
  Abs/1 -> Compare To Constant2/1, Stop/1
  Compare To Constant2/1 -> AND/3
  NOT1/1 -> AND/4
  BogieIsolated/1 -> AND1/2, NOT1/1
  AND1/1 -> SR Latch - Reset Priority/2  "TCUSlip"

== system TractionSystem/Traction (Per Vehicle)/MotorVehicle/VehicleTractionConvertersSystem/BogieTractionConverterSystem (Per Bogie)/TractionConverterSystem/TractionConverterMaxEffortPossible/MotorVehicle ==
  AxleHasMotor : Inport  Partition=on  PartitionDimension=1  PartitionWidth=1  PartitionOffset=0
  LinearWheelSpeed : Inport  Port=2  Partition=on  PartitionDimension=1  PartitionWidth=1  PartitionOffset=0
  AvailablePower : Inport  Port=3
  AvailableTorque : Inport  Port=4
  WheelRadius : Inport  Port=5
  MotorFailure : Inport  Port=6  Partition=on  PartitionDimension=1  PartitionWidth=1  PartitionOffset=0
  DBAvailable : Inport  Port=7
  For Each : ForEach  DisableCoverage=on
  If : If  IfExpression=u1
  Merge{,1..3} (4 alike) : Merge
  MotorAxle : Subsystem
  NoMotorAxle : Subsystem
  MaximumTractionEffortPossible : Outport  ConcatenationDimension=1
  MaxBrakingEffortPossible : Outport  Port=2  ConcatenationDimension=1
  MaxTractionPowerPossible : Outport  Port=3  ConcatenationDimension=1
  MaxBrakingPowerPossible : Outport  Port=4  ConcatenationDimension=1
  wires:
  LinearWheelSpeed/1 -> MotorAxle/1(LinearWheelSpeed)
  AvailablePower/1 -> MotorAxle/2(AvailablePower)
  AvailableTorque/1 -> MotorAxle/3(AvailableTorque)
  WheelRadius/1 -> MotorAxle/4(WheelRadius)
  MotorAxle/1(MaximumTractionEffortPossible) -> Merge1/1
  MotorAxle/2(MaximumBrakingEffortPossible) -> Merge/1
  AxleHasMotor/1 -> If/1
  If/2 -> NoMotorAxle/Action
  If/1 -> MotorAxle/Action
  Merge/1 -> MaxBrakingEffortPossible/1
  Merge1/1 -> MaximumTractionEffortPossible/1
  NoMotorAxle/1(MaximumTractionEffortPossible) -> Merge1/2
  NoMotorAxle/2(MaximumBrakingEffortPossible) -> Merge/2
  MotorFailure/1 -> MotorAxle/5(MotorFailure)
  DBAvailable/1 -> MotorAxle/6(DBAvailable)
  NoMotorAxle/4(MaximumBrakingPowerPossible) -> Merge2/2
  NoMotorAxle/3(MaximumTractionPowerPossible) -> Merge3/2
  Merge3/1 -> MaxTractionPowerPossible/1
  Merge2/1 -> MaxBrakingPowerPossible/1
  MotorAxle/4(MaximumBrakingPowerPossible) -> Merge2/1
  MotorAxle/3(MaximumTractionPowerPossible) -> Merge3/1

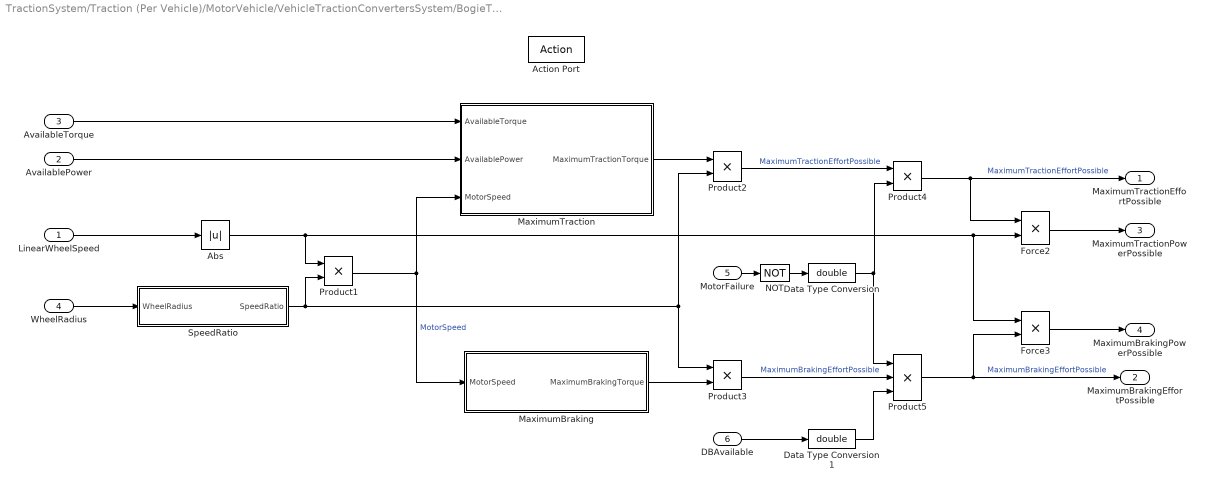
== system TractionSystem/Traction (Per Vehicle)/MotorVehicle/VehicleTractionConvertersSystem/BogieTractionConverterSystem (Per Bogie)/TractionConverterSystem/TractionConverterMaxEffortPossible/MotorVehicle/MotorAxle ==
  LinearWheelSpeed : Inport
  AvailablePower : Inport  Port=2
  AvailableTorque : Inport  Port=3
  WheelRadius : Inport  Port=4
  MotorFailure : Inport  Port=5
  DBAvailable : Inport  Port=6
  Action Port : ActionPort  ActionPortLabel=if(u1)
  Abs : Abs
  Data Type Conversion : DataTypeConversion  OutDataTypeStr=double
  Data Type Conversion1 : DataTypeConversion  OutDataTypeStr=double
  Force2 : Product  Inputs=**
  Force3 : Product  Inputs=**
  MaximumBraking : Subsystem
  MaximumTraction : Subsystem
  NOT : Logic  Operator=NOT  AllPortsSameDT=off  OutDataTypeStr=boolean
  Product{1..4} (4 alike) : Product
  Product5 : Product  Inputs=3
  SpeedRatio : Subsystem
  MaximumTractionEffortPossible : Outport
  MaximumBrakingEffortPossible : Outport  Port=2
  MaximumTractionPowerPossible : Outport  Port=3  VectorParamsAs1DForOutWhenUnconnected=off
  MaximumBrakingPowerPossible : Outport  Port=4  VectorParamsAs1DForOutWhenUnconnected=off
  wires:
  Product2/1 -> Product4/1  "MaximumTractionEffortPossible"
  AvailablePower/1 -> MaximumTraction/2(AvailablePower)
  AvailableTorque/1 -> MaximumTraction/1(AvailableTorque)
  Product1/1 -> MaximumTraction/3(MotorSpeed), MaximumBraking/1(MotorSpeed)  "MotorSpeed"
  MaximumTraction/1(MaximumTractionTorque) -> Product2/1
  SpeedRatio/1(SpeedRatio) -> Product1/2, Product3/1, Product2/2
  MaximumBraking/1(MaximumBrakingTorque) -> Product3/2
  WheelRadius/1 -> SpeedRatio/1(WheelRadius)
  Product3/1 -> Product5/2  "MaximumBrakingEffortPossible"
  Product4/1 -> Force2/1, MaximumTractionEffortPossible/1  "MaximumTractionEffortPossible"
  MotorFailure/1 -> NOT/1
  NOT/1 -> Data Type Conversion/1
  Data Type Conversion/1 -> Product5/1, Product4/2
  DBAvailable/1 -> Data Type Conversion1/1
  Data Type Conversion1/1 -> Product5/3
  Product5/1 -> MaximumBrakingEffortPossible/1, Force3/2  "MaximumBrakingEffortPossible"
  Force3/1 -> MaximumBrakingPowerPossible/1
  Force2/1 -> MaximumTractionPowerPossible/1
  LinearWheelSpeed/1 -> Abs/1
  Abs/1 -> Force3/1, Force2/2, Product1/1

== system TractionSystem/Traction (Per Vehicle)/MotorVehicle/VehicleTractionConvertersSystem/BogieTractionConverterSystem (Per Bogie)/TractionConverterSystem/TractionConverterMaxEffortPossible/MotorVehicle/NoMotorAxle ==
  Action Port : ActionPort  ActionPortLabel=else
  Constant{,1..3} (4 alike) : Constant  Value=0
  MaximumTractionEffortPossible : Outport
  MaximumBrakingEffortPossible : Outport  Port=2
  MaximumTractionPowerPossible : Outport  Port=3
  MaximumBrakingPowerPossible : Outport  Port=4
  wires:
  Constant1/1 -> MaximumBrakingEffortPossible/1  "MaximumBrakingEffortPossible"
  Constant/1 -> MaximumTractionEffortPossible/1  "MaximumTractionEffortPossible"
  Constant2/1 -> MaximumTractionPowerPossible/1  "MaximumTractionPowerPossible"
  Constant3/1 -> MaximumBrakingPowerPossible/1  "MaximumBrakingPowerPossible"

== system TractionSystem/Traction (Per Vehicle)/MotorVehicle/VehicleTractionConvertersSystem/BogieTractionConverterSystem (Per Bogie)/TractionConverterSystem/TractionConverterMaxEffortPossible/MotorVehicle/MotorAxle/MaximumBraking ==
  MotorSpeed : Inport
  Constant1 : Constant  Value=BrakingRatedTorque
  Constant2 : Constant  Value=BrakingDesignPower
  MinMax : MinMax  Inputs=2
  Pmax/v : Product  Inputs=*/
  RampUpCurve : TractionLib/BrakingTorque/CurveEquations/RampUpCurve  SystemSampleTime=-1  Latency=0  AutoFrameSizeCalculation=off
      settings: SourceProductName=Train Utilities
  safedivide : Saturate  UpperLimit=1e6  LowerLimit=eps
  MaximumBrakingTorque : Outport
  wires:
  safedivide/1 -> Pmax/v/2
  Pmax/v/1 -> MinMax/2  "ConstantPower"
  RampUpCurve/1 -> MinMax/1
  Constant1/1 -> RampUpCurve/1  "ConstantTorque"
  Constant2/1 -> Pmax/v/1
  MinMax/1 -> MaximumBrakingTorque/1  "MaximumBrakingTorque"
  MotorSpeed/1 -> RampUpCurve/2, safedivide/1

== system TractionSystem/Traction (Per Vehicle)/MotorVehicle/VehicleTractionConvertersSystem/BogieTractionConverterSystem (Per Bogie)/TractionConverterSystem/TractionConverterMaxEffortPossible/MotorVehicle/MotorAxle/MaximumTraction ==
  AvailableTorque : Inport
  AvailablePower : Inport  Port=2
  MotorSpeed : Inport  Port=3
  Constant1 : Constant  Value=TractionRatedTorque
  Constant2 : Constant  Value=TractionDesignPower
  MinMax : MinMax  Inputs=2
  Pmax/v : Product  Inputs=*/
  PowerAvailble : Product
  Saturation1 : Saturate  UpperLimit=1  LowerLimit=0
  Saturation3 : Saturate  UpperLimit=1  LowerLimit=0
  TorqueAvailable : Product
  safedivide : Saturate  UpperLimit=1e6  LowerLimit=eps
  MaximumTractionTorque : Outport
  wires:
  TorqueAvailable/1 -> MinMax/1
  AvailablePower/1 -> Saturation3/1
  Saturation1/1 -> TorqueAvailable/2
  PowerAvailble/1 -> Pmax/v/1
  safedivide/1 -> Pmax/v/2
  Saturation3/1 -> PowerAvailble/2
  Pmax/v/1 -> MinMax/2  "ConstantPower"
  Constant1/1 -> TorqueAvailable/1  "ConstantTorque"
  Constant2/1 -> PowerAvailble/1
  AvailableTorque/1 -> Saturation1/1
  MotorSpeed/1 -> safedivide/1
  MinMax/1 -> MaximumTractionTorque/1  "MaximumTractionTorque"

== system TractionSystem/Traction (Per Vehicle)/MotorVehicle/VehicleTractionConvertersSystem/BogieTractionConverterSystem (Per Bogie)/TractionConverterSystem/TractionConverterMaxEffortPossible/MotorVehicle/MotorAxle/SpeedRatio ==
  WheelRadius : Inport
  Constant : Constant  Value=GearRatio
  Pmax/v1 : Product  Inputs=*/
  safedivide1 : Saturate  UpperLimit=1e6  LowerLimit=eps
  SpeedRatio : Outport  VectorParamsAs1DForOutWhenUnconnected=off
  wires:
  Pmax/v1/1 -> SpeedRatio/1
  safedivide1/1 -> Pmax/v1/2
  WheelRadius/1 -> safedivide1/1
  Constant/1 -> Pmax/v1/1
